simulink model "Test_01"  (R2017b)
settings: Solver=ode45  StartTime=0.0  StopTime=8  RelTol=1e-3  EnableMultiTasking=on
values from neighbouring files (symbols this model uses):
  beta = beta (k)    [Parameter_2M_DFIG_and_BESS.m]
  Cbus = 80e-3    (= 0.08)    [Parameter_2M_DFIG_and_BESS.m]
  cp_opt_abs = abs(max(Cp))    [Parameter_2M_DFIG_and_BESS.m]
  D = 0.1    [Parameter_2M_DFIG_and_BESS.m]
  f = 60    [Parameter_2M_DFIG_and_BESS.m]
  Fs = 1.8    [Parameter_2M_DFIG_and_BESS.m]
  fsw = 4e3    (= 4000)    [Parameter_2M_DFIG_and_BESS.m]
  J = 90    [Parameter_2M_DFIG_and_BESS.m]
  ki_id = (wni^2)*Lr*sigma    (= 491.599501999)    [Parameter_2M_DFIG_and_BESS.m]
  ki_idg = (wnig^2)*Lg    (= 68.6450725305)    [Parameter_2M_DFIG_and_BESS.m]
  ki_iq = ki_id    (= 491.599501999)    [Parameter_2M_DFIG_and_BESS.m]
  ki_iqg = ki_idg    (= 68.6450725305)    [Parameter_2M_DFIG_and_BESS.m]
  ki_v = -300000    [Parameter_2M_DFIG_and_BESS.m]
  kp_id = (2*wni*sigma*Lr)-Rr    (= 0.5771)    [Parameter_2M_DFIG_and_BESS.m]
  kp_idg = (2*wnig*Lg)-Rg    (= 0.364153420404)    [Parameter_2M_DFIG_and_BESS.m]
  kp_iq = kp_id    (= 0.5771)    [Parameter_2M_DFIG_and_BESS.m]
  kp_iqg = kp_idg    (= 0.364153420404)    [Parameter_2M_DFIG_and_BESS.m]
  kp_v = -1000    [Parameter_2M_DFIG_and_BESS.m]
  Kpg = 1/(1.5*Vs*sqrt(2/3))    [Parameter_2M_DFIG_and_BESS.m]
  Kqg = -Kpg    [Parameter_2M_DFIG_and_BESS.m]
  lambda_opt = abs(lambda(posicion))    [Parameter_2M_DFIG_and_BESS.m]
  Lg = 483e-6    (= 0.000483)    [Parameter_2M_DFIG_and_BESS.m]
  Lm = 2.5e-3    (= 0.0025)    [Parameter_2M_DFIG_and_BESS.m]
  Lr = Lm + Lsr    (= 0.002587)    [Parameter_2M_DFIG_and_BESS.m]
  Ls = Lm + Lsi    (= 0.002587)    [Parameter_2M_DFIG_and_BESS.m]
  Lsi = 87e-6    (= 8.7e-05)    [Parameter_2M_DFIG_and_BESS.m]
  N = 100    [Parameter_2M_DFIG_and_BESS.m]
  p = 2    [Parameter_2M_DFIG_and_BESS.m]
  Ps = 2e6    (= 2000000)    [Parameter_2M_DFIG_and_BESS.m]
  Radio = 44    [Parameter_2M_DFIG_and_BESS.m]
  Rg = 20e-6    (= 2e-05)    [Parameter_2M_DFIG_and_BESS.m]
  ro = 1.225    [Parameter_2M_DFIG_and_BESS.m]
  Rr = 2.9e-3    (= 0.0029)    [Parameter_2M_DFIG_and_BESS.m]
  Rs = 2.6e-3    (= 0.0026)    [Parameter_2M_DFIG_and_BESS.m]
  sigma = 1- Lm^2/(Ls*Lr)    (= 0.0661284179513)    [Parameter_2M_DFIG_and_BESS.m]
  Ts = 1/fsw/f    (= 4.16666666667e-06)    [Parameter_2M_DFIG_and_BESS.m]
  Vbus_ref = 1200    [Parameter_2M_DFIG_and_BESS.m]
  Vdc_bat_ref = 1300    [Parameter_2M_DFIG_and_BESS.m]
  Vs = 690    [Parameter_2M_DFIG_and_BESS.m]
undefined symbols (not defined in the file or in its folder): D1, D11, Delta, DiscIntNeverNeededParam, Ion, Lithium
libraries: powerlib x60, powerlib_meascontrol x30, simulink x2, electricdrivelib x1, sps_avr x1
(part 2 of 2)

== system Test_01/BESS 1.0 MW 690 V/Bess Monitor ==
  note: BATTERY STORAGE SYSTEM
  note: Tip Speed Ratio
  note: Charging Power
  note: Discharging Power
  note: Id current control
  Mux{,13..15} (4 alike) : Mux  Inputs=2
  Scope3 : Scope  NumInputPorts=6
  wires:
  [P_bat_ref] -> Mux14/1
  [V_dc_bat] -> Mux/2
  Mux13/1 -> Scope3/2  "Charging Power (W)"
  [P_SOC_ref] -> Mux13/1
  [P_bat] -> Mux14/2, Mux13/2
  [id_bat_ref] -> Mux15/1
  [V_dc_bat_ref] -> Mux/1
  Mux/1 -> Scope3/1  "Vbus* / Vbus (V)"
  [id_bat] -> Mux15/2
  Mux14/1 -> Scope3/3  "Discharging Power (W)"
  [SOC] -> Scope3/5  "SOC (%)"
  [I_dc_bat] -> Scope3/4  "Battery Current (Amp)"
  Mux15/1 -> Scope3/6  "Id*/Id (Amp)"

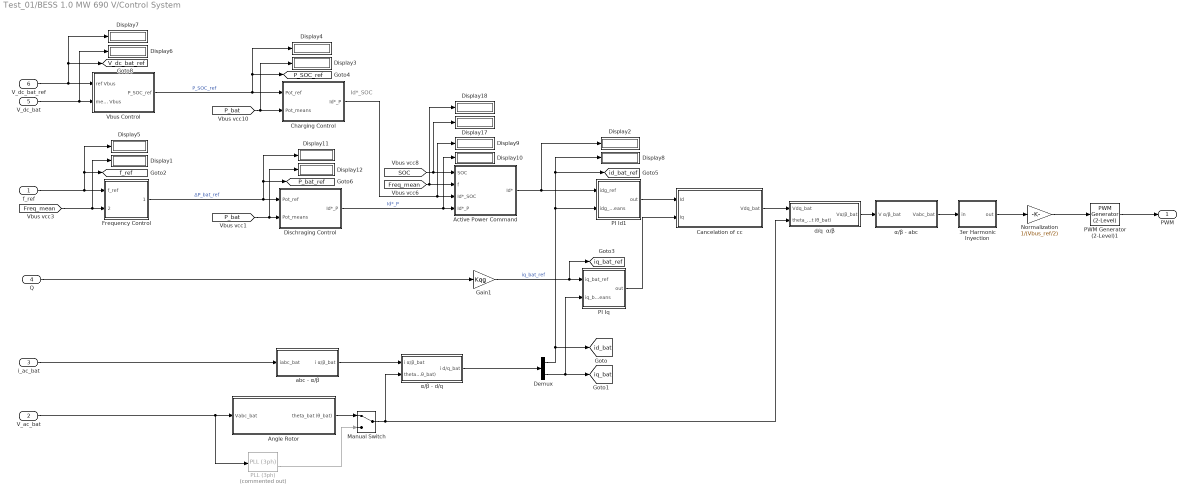
== system Test_01/BESS 1.0 MW 690 V/Control System ==
  note: Id*_SOC
  f_ref : Inport
  "V_ac_bat " : Inport  Port=2
  i_ac_bat : Inport  Port=3
  Q : Inport  Port=4
  V_dc_bat : Inport  Port=5
  V_dc_bat_ref : Inport  Port=6
  " Angle Rotor" : Subsystem
  3er Harmonic Inyection : Subsystem
  Active Power Command : Subsystem
  Cancelation of cc : Subsystem
  Charging Control : Subsystem
  Demux : Demux  Outputs=2
  Dischraging Control : Subsystem
  Display{1..12,17..18} (14 alike) : Display
  Frequency Control : Subsystem
  Gain1 : Gain  Gain=Kqg
  Manual Switch : ManualSwitch
  Normalization : Gain  Gain=1/(Vbus_ref/2)
  PI Id1 : Subsystem
  PI Iq : Subsystem
  PLL (3ph) : powerlib_meascontrol/PLL/PLL (3ph)  Commented=on  Fmin=45  Par_Init=[0, 60]  ParK=[180, 3200, 1]  TcD=1e-4  MaxRateChangeFreq=12  FilterCutOffFreq=25  Ts=0  AGC=on
      link override Model/abc to dq0: Alignment=Aligned with phase A axis
  PWM Generator (2-Level)1 : powerlib_meascontrol/Pulse & Signal Generators/PWM Generator (2-Level)  ModulatorType=Three-phase bridge (6 pulses)  ModulatorMode=Unsynchronized  Fc=fsw  Pc=0  nF=27  MinMax="[ -1  1 ]"  SamplingTechnique=Natural  ModulatingSignals=off  m=0.8  Freq=60  Phase=0  Ts=0  ShowCarrierOutport=off
      settings: SourceProductName=Simscape Power Systems
  Vbus Control : Subsystem
  "abc - α/β  " : Subsystem
  "d/q  α/β " : Subsystem
  α/β - abc : Subsystem
  α/β - d/q : Subsystem
  PWM : Outport
  tag scope: P_SOC_ref=global, P_bat_ref=global, V_dc_bat_ref=global, f_ref=global, id_bat=global, id_bat_ref=global, iq_bat=global, iq_bat_ref=global
  wires:
  PWM Generator (2-Level)1/1 -> PWM/1
  PLL (3ph)/2 -> Manual Switch/2
  α/β - d/q/1(i d/q_bat) -> Demux/1
  Manual Switch/1 -> "d/q  α/β "/2(theta_bat (θ_bat)), α/β - d/q/2(theta_bat (θ_bat))
  " Angle Rotor"/1(theta_bat (θ_bat)) -> Manual Switch/1
  "V_ac_bat "/1 -> PLL (3ph)/1, " Angle Rotor"/1(Vabc_bat)
  α/β - abc/1(Vabc_bat) -> 3er Harmonic Inyection/1(in)
  i_ac_bat/1 -> "abc - α/β  "/1(iabc_bat)
  "d/q  α/β "/1("Vα/β_bat ") -> α/β - abc/1(V α/β_bat)
  "abc - α/β  "/1(i α/β_bat) -> α/β - d/q/1(i α/β_bat)
  3er Harmonic Inyection/1(out) -> Normalization/1
  PI Id1/1(out) -> Cancelation of cc/1(Id)
  PI Iq/1("out ") -> Cancelation of cc/2(Iq)
  Demux/2 -> [iq_bat], PI Iq/2(iq_bat_means)
  Gain1/1 -> [iq_bat_ref], PI Iq/1(iq_bat_ref)  "iq_bat_ref"
  Cancelation of cc/1(" Vdq_bat") -> "d/q  α/β "/1(Vdq_bat)
  Normalization/1 -> PWM Generator (2-Level)1/1
  Frequency Control/1("ΔP_bat_ref ") -> [P_bat_ref], Display11/1, Dischraging Control/1("Pot_ref ")  "ΔP_bat_ref"
  V_dc_bat/1 -> Display6/1, Vbus Control/2("means Vbus ")
  f_ref/1 -> Frequency Control/1(f_ref), [f_ref], Display5/1
  Q/1 -> Gain1/1
  [P_bat] -> Display12/1, Dischraging Control/2("Pot_means ")
  [Freq_mean] -> Display1/1, Frequency Control/2(f_means)
  Demux/1 -> PI Id1/2(idg_means), Display8/1, [id_bat_ref], [id_bat]
  [Freq_mean] -> Active Power Command/2(f), Display18/1
  [SOC] -> Active Power Command/1(SOC), Display17/1
  V_dc_bat_ref/1 -> [V_dc_bat_ref], Display7/1, Vbus Control/1("ref Vbus ")
  Active Power Command/1(Id*) -> Display2/1, PI Id1/1(idg_ref)
  Dischraging Control/1(Id*_P) -> Display10/1, Active Power Command/4(Id*_P)  "Id*_P"
  Charging Control/1(Id*_P) -> Display9/1, Active Power Command/3(Id*_SOC)
  Vbus Control/1(P_SOC_ref) -> [P_SOC_ref], Display4/1, Charging Control/1("Pot_ref ")  "P_SOC_ref"
  [P_bat] -> Charging Control/2("Pot_means "), Display3/1

== system Test_01/BESS 1.0 MW 690 V/Measurement of Power - Frequency ==
  PLL (3ph)1 : powerlib_meascontrol/PLL/PLL (3ph)  Fmin=45  Par_Init=[0, f]  ParK=[180, 3200, 1]  TcD=1e-4  MaxRateChangeFreq=12  FilterCutOffFreq=25  Ts=0  AGC=on
  "Power (3ph, Instantaneous)1" : powerlib_meascontrol/Measurements/Power (3ph, Instantaneous)
      settings: SourceProductName=Simscape Power Systems
  F (Hz) : Outport
  P (W) : Outport  Port=2
  Q (VAR) : Outport  Port=3
  tag scope: Freq_mean=global, P_bat=global, Q_bat=global
  wires:
  [V_ac_bat] -> "Power (3ph, Instantaneous)1"/1, PLL (3ph)1/1
  "Power (3ph, Instantaneous)1"/1 -> P (W)/1, [P_bat]  "Pot"
  PLL (3ph)1/1 -> F (Hz)/1, [Freq_mean]
  [I_ac_bat] -> "Power (3ph, Instantaneous)1"/2
  "Power (3ph, Instantaneous)1"/2 -> Q (VAR)/1, [Q_bat]

== system Test_01/BESS 1.0 MW 690 V/Subsystem1 ==
  In1 : Inport
  Bus Selector : BusSelector  OutputSignals=SOC (%),Current (A),Voltage (V)
  tag scope: I_dc_bat=global, SOC=global, V_dc_bat=global
  wires:
  Bus Selector/3 -> [V_dc_bat]  "<Voltage (V)>"
  Bus Selector/1 -> [SOC]  "<SOC (%)>"
  In1/1 -> Bus Selector/1
  Bus Selector/2 -> [I_dc_bat]  "<Current (A)>"

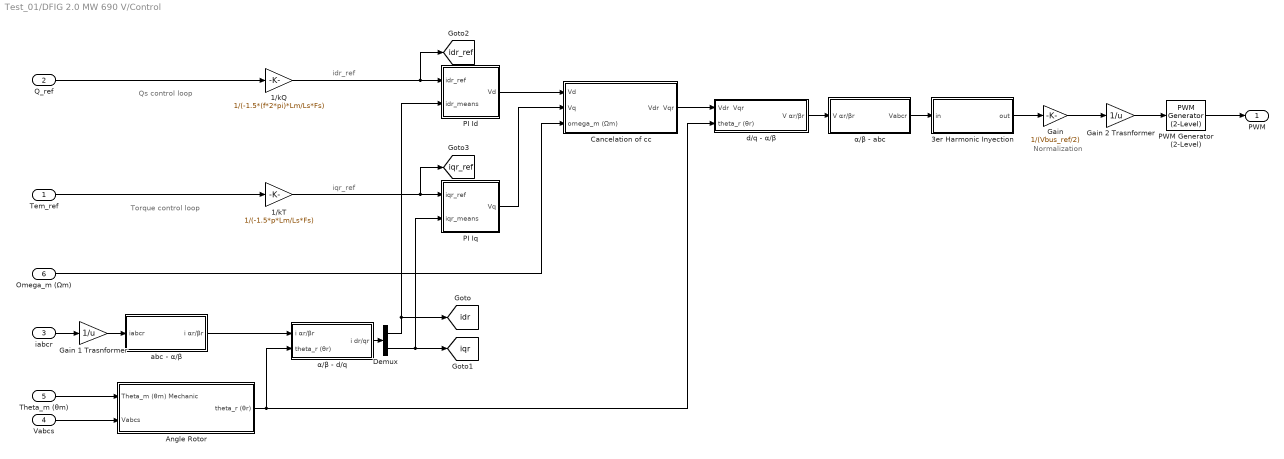
== system Test_01/DFIG 2.0 MW 690 V/Control ==
  note: Normalization
  note: Torque control loop
  note: iqr_ref
  note: idr_ref
  note: Qs control loop
  Tem_ref : Inport
  Q_ref : Inport  Port=2
  iabcr : Inport  Port=3
  Vabcs : Inport  Port=4
  Theta_m (θm) : Inport  Port=5
  "Omega_m (Ωm) " : Inport  Port=6
  " Angle Rotor" : Subsystem
  1/kQ : Gain  Gain=1/(-1.5*(f*2*pi)*Lm/Ls*Fs)
  1/kT : Gain  Gain=1/(-1.5*p*Lm/Ls*Fs)
  3er Harmonic Inyection : Subsystem
  Cancelation of cc : Subsystem
  Demux : Demux  Outputs=2
  Gain : Gain  Gain=1/(Vbus_ref/2)
  Gain 1 Trasnformer : Gain  Gain=1/u
  Gain 2 Trasnformer : Gain  Gain=1/u
  PI Id : Subsystem
  PI Iq : Subsystem
  PWM Generator (2-Level) : powerlib_meascontrol/Pulse & Signal Generators/PWM Generator (2-Level)  ModulatorType=Three-phase bridge (6 pulses)  ModulatorMode=Unsynchronized  Fc=fsw  Pc=0  nF=27  MinMax="[ -1  1 ]"  SamplingTechnique=Natural  ModulatingSignals=off  m=0.8  Freq=60  Phase=0  Ts=0  ShowCarrierOutport=off
      settings: SourceProductName=Simscape Power Systems
  "abc - α/β " : Subsystem
  d/q - α/β : Subsystem
  α/β - abc : Subsystem
  α/β - d/q : Subsystem
  PWM : Outport
  tag scope: idr=global, idr_ref=global, iqr=global, iqr_ref=global
  wires:
  α/β - abc/1(Vabcr) -> 3er Harmonic Inyection/1(in)
  d/q - α/β/1(V αr/βr) -> α/β - abc/1(V αr/βr)
  iabcr/1 -> Gain 1 Trasnformer/1
  "abc - α/β "/1(i αr/βr) -> α/β - d/q/1(i αr/βr)
  3er Harmonic Inyection/1(out) -> Gain/1
  Theta_m (θm)/1 -> " Angle Rotor"/1(Theta_m (θm) Mechanic)
  Vabcs/1 -> " Angle Rotor"/2(Vabcs)
  " Angle Rotor"/1(theta_r (θr)) -> d/q - α/β/2(theta_r (θr)), α/β - d/q/2(theta_r (θr))
  PI Id/1(Vd) -> Cancelation of cc/1(Vd)
  PI Iq/1(Vq) -> Cancelation of cc/2(Vq)
  α/β - d/q/1(i dr/qr) -> Demux/1
  Demux/2 -> PI Iq/2(iqr_means), [iqr]
  Demux/1 -> PI Id/2(idr_means), [idr]
  1/kT/1 -> [iqr_ref], PI Iq/1(iqr_ref)
  Q_ref/1 -> 1/kQ/1
  Cancelation of cc/1(Vdr  Vqr) -> d/q - α/β/1(Vdr  Vqr)
  Gain/1 -> Gain 2 Trasnformer/1
  Gain 1 Trasnformer/1 -> "abc - α/β "/1(iabcr)
  Gain 2 Trasnformer/1 -> PWM Generator (2-Level)/1
  PWM Generator (2-Level)/1 -> PWM/1
  Tem_ref/1 -> 1/kT/1
  "Omega_m (Ωm) "/1 -> Cancelation of cc/3(omega_m (Ωm))
  1/kQ/1 -> [idr_ref], PI Id/1(idr_ref)

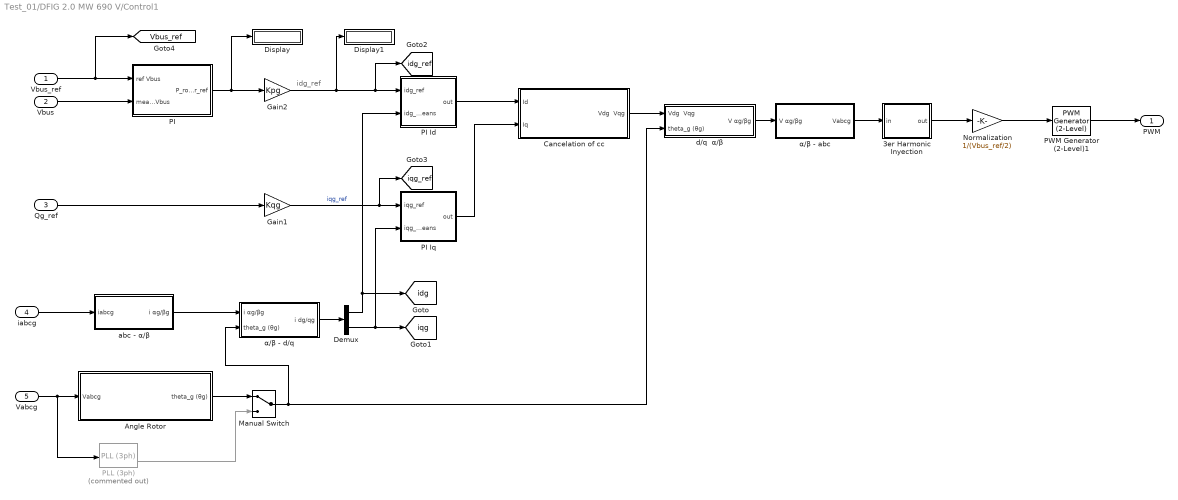
== system Test_01/DFIG 2.0 MW 690 V/Control1 ==
  note: idg_ref
  Vbus_ref : Inport
  Vbus : Inport  Port=2
  Qg_ref : Inport  Port=3
  iabcg : Inport  Port=4
  "Vabcg " : Inport  Port=5
  " Angle Rotor" : Subsystem
  3er Harmonic Inyection : Subsystem
  Cancelation of cc : Subsystem
  Demux : Demux  Outputs=2
  Display : Display
  Display1 : Display
  Gain1 : Gain  Gain=Kqg
  Gain2 : Gain  Gain=Kpg
  Manual Switch : ManualSwitch
  Normalization : Gain  Gain=1/(Vbus_ref/2)
  PI : Subsystem
  PI Id : Subsystem
  PI Iq : Subsystem
  PLL (3ph) : powerlib_meascontrol/PLL/PLL (3ph)  Commented=on  Fmin=45  Par_Init=[0, 60]  ParK=[180, 3200, 1]  TcD=1e-4  MaxRateChangeFreq=12  FilterCutOffFreq=25  Ts=0  AGC=on
      link override Model/abc to dq0: Alignment=Aligned with phase A axis
  PWM Generator (2-Level)1 : powerlib_meascontrol/Pulse & Signal Generators/PWM Generator (2-Level)  ModulatorType=Three-phase bridge (6 pulses)  ModulatorMode=Unsynchronized  Fc=fsw  Pc=0  nF=27  MinMax="[ -1  1 ]"  SamplingTechnique=Natural  ModulatingSignals=off  m=0.8  Freq=60  Phase=0  Ts=0  ShowCarrierOutport=off
      settings: SourceProductName=Simscape Power Systems
  "abc - α/β  " : Subsystem
  "d/q  α/β " : Subsystem
  α/β - abc : Subsystem
  α/β - d/q : Subsystem
  PWM : Outport
  tag scope: Vbus_ref=global, idg=global, idg_ref=global, iqg=global, iqg_ref=global
  wires:
  Normalization/1 -> PWM Generator (2-Level)1/1
  Cancelation of cc/1(Vdg  Vqg) -> "d/q  α/β "/1(Vdg  Vqg)
  Gain1/1 -> PI Iq/1(iqg_ref), [iqg_ref]  "iqg_ref"
  Demux/1 -> PI Id/2(idg_means), [idg]
  Demux/2 -> PI Iq/2(iqg_means), [iqg]
  PI Iq/1(out) -> Cancelation of cc/2(Iq)
  PI Id/1(out) -> Cancelation of cc/1(Id)
  3er Harmonic Inyection/1(out) -> Normalization/1
  "abc - α/β  "/1(i αg/βg) -> α/β - d/q/1(i αg/βg)
  "d/q  α/β "/1(V αg/βg) -> α/β - abc/1(V αg/βg)
  iabcg/1 -> "abc - α/β  "/1(iabcg)
  Vbus_ref/1 -> [Vbus_ref], PI/1("ref Vbus ")
  Gain2/1 -> Display1/1, [idg_ref], PI Id/1(idg_ref)
  Vbus/1 -> PI/2("means Vbus ")
  Qg_ref/1 -> Gain1/1
  α/β - abc/1(Vabcg) -> 3er Harmonic Inyection/1(in)
  "Vabcg "/1 -> " Angle Rotor"/1("Vabcg "), PLL (3ph)/1
  PI/1(P_rotor_ref) -> Display/1, Gain2/1
  " Angle Rotor"/1(theta_g (θg)) -> Manual Switch/1
  Manual Switch/1 -> "d/q  α/β "/2(theta_g (θg)), α/β - d/q/2(theta_g (θg))
  α/β - d/q/1(i dg/qg) -> Demux/1
  PLL (3ph)/2 -> Manual Switch/2
  PWM Generator (2-Level)1/1 -> PWM/1

== system Test_01/DFIG 2.0 MW 690 V/MPPT ==
  note: Zone 2: MPPT with Vw 5 - 11
  Omega_m : Inport
  Display1 : Display
  Display2 : Display
  Gearbox Ratio Generator Torque (-)1 : Gain  Gain=-1/N
  Gearbox Ratio1 : Gain  Gain=1/N
  Kopt : Gain  Gain=0.5*ro*pi*(Radio)^5/(lambda_opt)^3*cp_opt_abs
  Product2 : Product  Inputs=**  SaturateOnIntegerOverflow=on  InputSameDT=on  OutDataTypeStr=Inherit: Same as first input
  omega^2 : Fcn  Expr=(u[1])^2
  Tem_ref : Outport
  "Pot_ref " : Outport  Port=2
  wires:
  Gearbox Ratio1/1 -> Product2/2, omega^2/1
  omega^2/1 -> Kopt/1
  Kopt/1 -> Product2/1, Gearbox Ratio Generator Torque (-)1/1
  Product2/1 -> "Pot_ref "/1, Display1/1  "Pt"
  Gearbox Ratio Generator Torque (-)1/1 -> Display2/1, Tem_ref/1
  Omega_m/1 -> Gearbox Ratio1/1

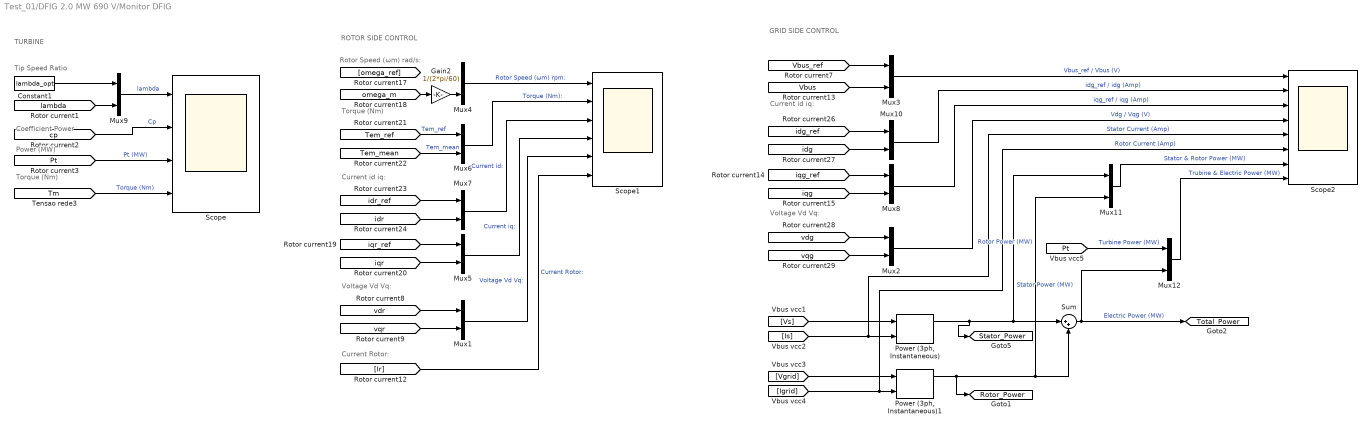
== system Test_01/DFIG 2.0 MW 690 V/Monitor DFIG ==
  note: ROTOR SIDE CONTROL
  note: Torque (Nm)
  note: Current id iq:
  note: Rotor Speed (ωm) rad/s:
  note: Voltage Vd Vq:
  note: TURBINE
  note: Torque (Nm)
  note: Power (MW)
  note: Coefficient Power
  note: Tip Speed Ratio
  note: GRID SIDE CONTROL
  note: Current id iq:
  note: Voltage Vd Vq:
  note: Current Rotor:
  Constant1 : Constant  Value=lambda_opt
  Gain2 : Gain  Gain=1/(2*pi/60)
  Mux{1..12} (12 alike) : Mux  Inputs=2
  "Power (3ph, Instantaneous)" : powerlib_meascontrol/Measurements/Power (3ph, Instantaneous)
      settings: SourceProductName=Simscape Power Systems
  "Power (3ph, Instantaneous)1" : powerlib_meascontrol/Measurements/Power (3ph, Instantaneous)
      settings: SourceProductName=Simscape Power Systems
  Scope : Scope  NumInputPorts=4
  Scope1 : Scope  NumInputPorts=6
  Scope2 : Scope  NumInputPorts=8
  Sum : Sum  Inputs=|++
  tag scope: Rotor_Power=global, Stator_Power=global, Total_Power=global
  wires:
  [iqr_ref] -> Mux5/1
  [iqr] -> Mux5/2
  [idr] -> Mux7/2
  [idr_ref] -> Mux7/1
  [vdr] -> Mux1/1
  [vqr] -> Mux1/2
  [vqg] -> Mux2/2
  [vdg] -> Mux2/1
  [idg_ref] -> Mux10/1
  [idg] -> Mux10/2
  [iqg] -> Mux8/2
  [iqg_ref] -> Mux8/1
  [Tem_ref] -> Mux6/1  "Tem_ref"
  [Vbus] -> Mux3/2
  [Vbus_ref] -> Mux3/1
  [cp] -> Scope/2  "Cp"
  [Pt] -> Scope/3  "Pt (MW)"
  [Tm] -> Scope/4  "Torque (Nm)"
  Mux4/1 -> Scope1/1  "Rotor Speed (ωm) rpm:"
  Mux6/1 -> Scope1/2  "Torque (Nm):"
  Mux7/1 -> Scope1/3  "Current id:"
  Mux5/1 -> Scope1/4  "Current iq:"
  Mux1/1 -> Scope1/5  "Voltage Vd Vq:"
  [Ir] -> Scope1/6  "Current Rotor:"
  [omega_m] -> Gain2/1
  Gain2/1 -> Mux4/2
  Mux3/1 -> Scope2/1  "Vbus_ref / Vbus (V)"
  Mux10/1 -> Scope2/2  "idg_ref / idg (Amp)"
  Mux8/1 -> Scope2/3  "iqg_ref / iqg (Amp)"
  Mux2/1 -> Scope2/4  "Vdg / Vqg (V)"
  [lambda] -> Mux9/2
  Constant1/1 -> Mux9/1
  Mux9/1 -> Scope/1  "lambda"
  [Tem_mean] -> Mux6/2  "Tem_mean"
  [Vs] -> "Power (3ph, Instantaneous)"/1
  [Vgrid] -> "Power (3ph, Instantaneous)1"/1
  [Igrid] -> "Power (3ph, Instantaneous)1"/2, Scope2/6  "Rotor Current (Amp)"
  [Is] -> "Power (3ph, Instantaneous)"/2, Scope2/5  "Stator Current (Amp)"
  "Power (3ph, Instantaneous)"/1 -> [Stator_Power], Mux11/1, Sum/1  "Stator Power (MW)"
  "Power (3ph, Instantaneous)1"/1 -> [Rotor_Power], Sum/2, Mux11/2  "Rotor Power (MW)"
  Sum/1 -> [Total_Power], Mux12/2  "Electric Power (MW)"
  Mux11/1 -> Scope2/7  "Stator & Rotor Power (MW)"
  [Pt] -> Mux12/1  "Turbine Power (MW)"
  Mux12/1 -> Scope2/8  "Trubine & Electric Power (MW)"

== system Test_01/DFIG 2.0 MW 690 V/Subsystem ==
  In1 : Inport
  Bus Selector : BusSelector  OutputSignals=Mechanical.Rotor angle thetam (rad),Mechanical.Rotor speed (wm),Mechanical.Electromagnetic torque Te (N*m)
  tag scope: Tem_mean=global, omega_m=global, tita_m=global
  wires:
  Bus Selector/2 -> [omega_m]  "<Rotor speed (wm)>"
  In1/1 -> Bus Selector/1
  Bus Selector/1 -> [tita_m]  "<Rotor angle thetam (rad)>"
  Bus Selector/3 -> [Tem_mean]  "<Electromagnetic torque Te (N*m)>"

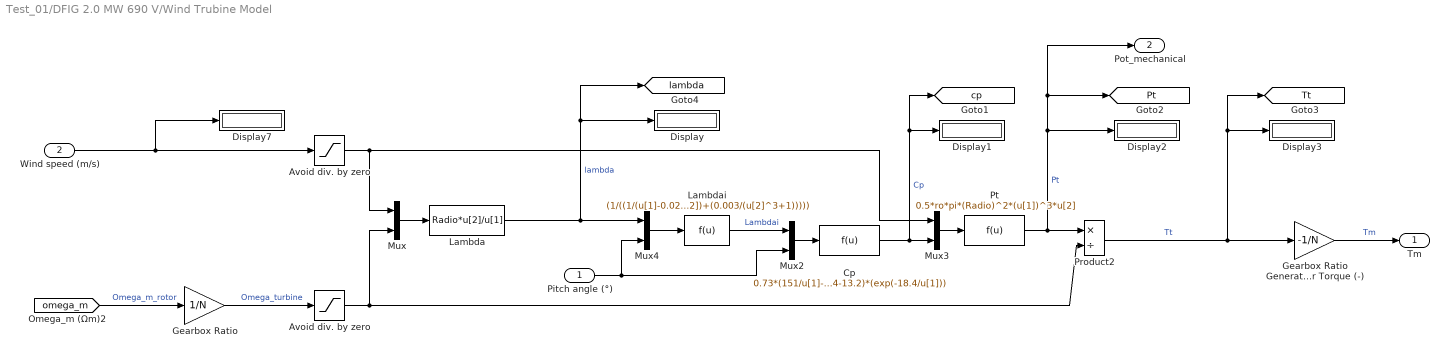
== system Test_01/DFIG 2.0 MW 690 V/Wind Trubine Model ==
  Pitch angle (°) : Inport
  Wind speed (m/s) : Inport  Port=2
  Avoid div. by zero : Saturate  UpperLimit=inf  LowerLimit=eps
  "Avoid div. by zero " : Saturate  UpperLimit=inf  LowerLimit=eps
  Cp : Fcn  Expr=0.73*(151/u[1]-0.58*u[2]-0.002*u[2]^2.14-13.2)*(exp(-18.4/u[1]))
  Display{,1..3,7} (5 alike) : Display
  Gearbox Ratio : Gain  Gain=1/N
  Gearbox Ratio Generator Torque (-) : Gain  Gain=-1/N
  Lambda : Fcn  Expr=Radio*u[2]/u[1]
  Lambdai : Fcn  Expr=(1/((1/(u[1]-0.02*u[2])+(0.003/(u[2]^3+1)))))
  Mux{,2..4} (4 alike) : Mux  Inputs=2
  Product2 : Product  Inputs=*/  SaturateOnIntegerOverflow=on  InputSameDT=on  OutDataTypeStr=Inherit: Same as first input
  Pt : Fcn  Expr=0.5*ro*pi*(Radio)^2*(u[1])^3*u[2]
  Tm : Outport
  Pot_mechanical : Outport  Port=2
  tag scope: Pt=global, Tt=global, cp=global, lambda=global
  wires:
  "Avoid div. by zero "/1 -> Product2/2, Mux/2
  Avoid div. by zero/1 -> Mux/1, Mux3/1
  [omega_m] -> Gearbox Ratio/1  "Omega_m_rotor"
  Mux3/1 -> Pt/1
  Cp/1 -> Display1/1, [cp], Mux3/2  "Cp"
  Mux/1 -> Lambda/1
  Mux2/1 -> Cp/1
  Product2/1 -> Display3/1, [Tt], Gearbox Ratio Generator Torque (-)/1  "Tt"
  Pt/1 -> Display2/1, Pot_mechanical/1, [Pt], Product2/1  "Pt"
  Gearbox Ratio/1 -> "Avoid div. by zero "/1  "Omega_turbine"
  Wind speed (m/s)/1 -> Display7/1, Avoid div. by zero/1
  Lambdai/1 -> Mux2/1  "Lambdai"
  Mux4/1 -> Lambdai/1
  Gearbox Ratio Generator Torque (-)/1 -> Tm/1  "Tm"
  Pitch angle (°)/1 -> Mux2/2, Mux4/2
  Lambda/1 -> Display/1, [lambda], Mux4/1  "lambda"

== system Test_01/Subsystem/Measurement of Power - Frequency1 ==
  PLL (3ph)1 : powerlib_meascontrol/PLL/PLL (3ph)  Fmin=45  Par_Init=[0, f]  ParK=[180, 3200, 1]  TcD=1e-4  MaxRateChangeFreq=12  FilterCutOffFreq=25  Ts=0  AGC=on
  "Power (3ph, Instantaneous)1" : powerlib_meascontrol/Measurements/Power (3ph, Instantaneous)
      settings: SourceProductName=Simscape Power Systems
  F (Hz) : Outport
  P (W) : Outport  Port=2
  wires:
  [I_ac_syn_low1] -> "Power (3ph, Instantaneous)1"/2
  PLL (3ph)1/1 -> F (Hz)/1
  "Power (3ph, Instantaneous)1"/1 -> P (W)/1  "Pot"
  [V_ac_syn_low1] -> PLL (3ph)1/1, "Power (3ph, Instantaneous)1"/1

== system Test_01/Subsystem/Measurement of Power - Frequency2 ==
  PLL (3ph)1 : powerlib_meascontrol/PLL/PLL (3ph)  Fmin=45  Par_Init=[0, f]  ParK=[180, 3200, 1]  TcD=1e-4  MaxRateChangeFreq=12  FilterCutOffFreq=25  Ts=0  AGC=on
  "Power (3ph, Instantaneous)1" : powerlib_meascontrol/Measurements/Power (3ph, Instantaneous)
      settings: SourceProductName=Simscape Power Systems
  F (Hz) : Outport
  P (W) : Outport  Port=2
  wires:
  [I_ac_syn_low2] -> "Power (3ph, Instantaneous)1"/2
  PLL (3ph)1/1 -> F (Hz)/1
  "Power (3ph, Instantaneous)1"/1 -> P (W)/1  "Pot"
  [V_ac_syn_low2] -> PLL (3ph)1/1, "Power (3ph, Instantaneous)1"/1

== system Test_01/BESS 1.0 MW 690 V/Control System/ Angle Rotor ==
  note: V α/β_bat
  Vabc_bat : Inport
  " abc - αβ " : Subsystem
  Demux : Demux  Outputs=2
  θv=tan^(-1) (Vβ/Vα) : Trigonometry  Operator=atan2
  theta_bat (θ_bat) : Outport
  wires:
  θv=tan^(-1) (Vβ/Vα)/1 -> theta_bat (θ_bat)/1
  Vabc_bat/1 -> " abc - αβ "/1(Vabc_bat)
  Demux/2 -> θv=tan^(-1) (Vβ/Vα)/1
  Demux/1 -> θv=tan^(-1) (Vβ/Vα)/2
  " abc - αβ "/1("V α/β_bat ") -> Demux/1

== system Test_01/BESS 1.0 MW 690 V/Control System/3er Harmonic Inyection ==
  in : Inport
  Gain : Gain  Gain=-0.5
  MinMax : MinMax
  MinMax1 : MinMax  Function=max
  Scope : Scope
  Sum : Sum  Inputs=|++
  Sum1 : Sum  Inputs=|++
  out : Outport
  wires:
  in/1 -> Sum1/1, MinMax1/1, MinMax/1
  MinMax/1 -> Sum/1
  MinMax1/1 -> Sum/2
  Sum1/1 -> out/1
  Sum/1 -> Gain/1
  Gain/1 -> Scope/1, Sum1/2

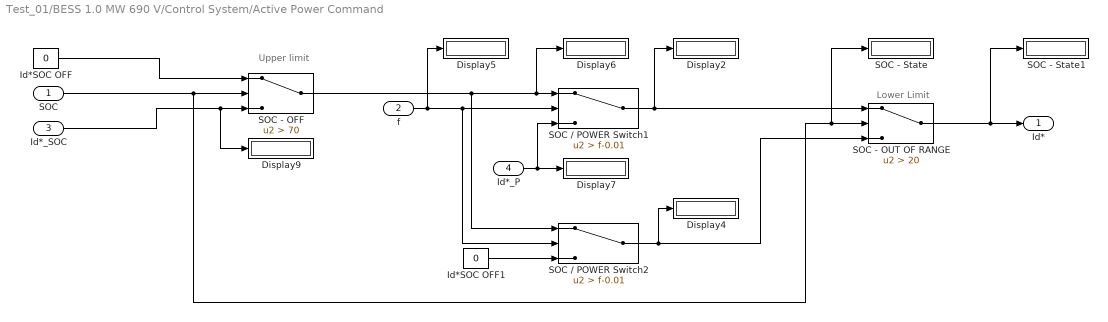
== system Test_01/BESS 1.0 MW 690 V/Control System/Active Power Command ==
  note: Lower Limit
  note: Upper limit
  SOC : Inport
  f : Inport  Port=2
  Id*_SOC : Inport  Port=3
  Id*_P : Inport  Port=4
  Display{2,4..7,9} (6 alike) : Display
  Id*SOC OFF : Constant  Value=0
  Id*SOC OFF1 : Constant  Value=0
  SOC - OFF : Switch  Criteria=u2 > Threshold  Threshold=70
  SOC - OUT OF RANGE : Switch  Criteria=u2 > Threshold  Threshold=20
  SOC - State : Display
  SOC - State1 : Display
  SOC / POWER Switch1 : Switch  Criteria=u2 > Threshold  Threshold=f-0.01
  SOC / POWER Switch2 : Switch  Criteria=u2 > Threshold  Threshold=f-0.01
  Id* : Outport
  wires:
  SOC / POWER Switch1/1 -> SOC - OUT OF RANGE/1, Display2/1
  f/1 -> Display5/1, SOC / POWER Switch2/2, SOC / POWER Switch1/2
  Id*_P/1 -> SOC / POWER Switch1/3, Display7/1
  SOC - OFF/1 -> SOC / POWER Switch2/1, SOC / POWER Switch1/1, Display6/1
  Id*SOC OFF/1 -> SOC - OFF/1
  Id*_SOC/1 -> Display9/1, SOC - OFF/3
  SOC / POWER Switch2/1 -> Display4/1, SOC - OUT OF RANGE/3
  SOC - OUT OF RANGE/1 -> SOC - State1/1, Id*/1
  Id*SOC OFF1/1 -> SOC / POWER Switch2/3
  SOC/1 -> SOC - State/1, SOC - OUT OF RANGE/2, SOC - OFF/2

== system Test_01/BESS 1.0 MW 690 V/Control System/Cancelation of cc ==
  Id : Inport
  Iq : Inport  Port=2
  Display : Display
  Fcn : Fcn  Expr=u[1]-u[4]*Lg*(2*pi*f)
  Fcn1 : Fcn  Expr=u[2]+u[3]*Lg*(2*pi*f)
  Mux : Mux  Inputs=2
  Mux1 : Mux
  " Vdq_bat" : Outport
  tag scope: vd_bat=global, vq_bat=global
  wires:
  Mux/1 -> " Vdq_bat"/1
  Fcn/1 -> [vd_bat], Display/1, Mux/1
  Fcn1/1 -> [vq_bat], Mux/2
  Id/1 -> Mux1/1
  Iq/1 -> Mux1/2
  Mux1/1 -> Fcn1/1, Fcn/1
  [id_bat] -> Mux1/3
  [iq_bat] -> Mux1/4

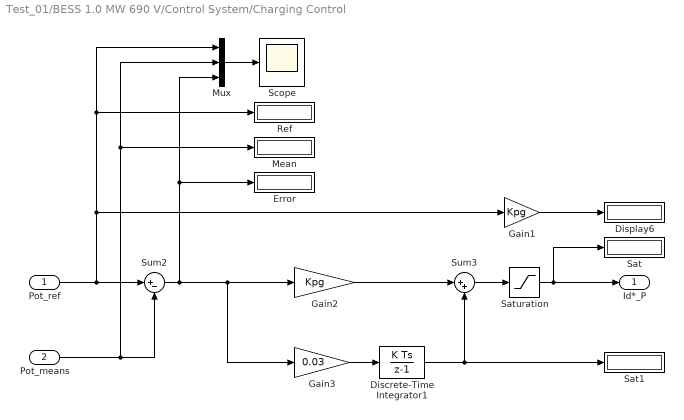
== system Test_01/BESS 1.0 MW 690 V/Control System/Charging Control ==
  "Pot_ref " : Inport
  "Pot_means " : Inport  Port=2
  Discrete-Time Integrator1 : DiscreteIntegrator  gainval=1  SampleTime=1/fsw  LimitOutput=on  UpperSaturationLimit=1200  LowerSaturationLimit=-1200  ICPrevOutput=DiscIntNeverNeededParam  ICPrevScaledInput=DiscIntNeverNeededParam
  Display6 : Display
  Error : Display
  Gain1 : Gain  Gain=Kpg
  Gain2 : Gain  Gain=Kpg
  Gain3 : Gain  Gain=0.03
  Mean : Display
  Mux : Mux  Inputs=3
  Ref : Display
  Sat : Display
  Sat1 : Display
  Saturation : Saturate  UpperLimit=1200  LowerLimit=-1200
  Scope : Scope
  Sum2 : Sum  Inputs=|+-
  Sum3 : Sum  Inputs=|++
  Id*_P : Outport
  wires:
  Sum2/1 -> Error/1, Mux/3, Gain2/1, Gain3/1
  Gain1/1 -> Display6/1
  Gain2/1 -> Sum3/1
  Sum3/1 -> Saturation/1
  Gain3/1 -> Discrete-Time Integrator1/1
  Discrete-Time Integrator1/1 -> Sat1/1, Sum3/2
  Mux/1 -> Scope/1
  "Pot_ref "/1 -> Mux/1, Ref/1, Gain1/1, Sum2/1
  "Pot_means "/1 -> Mux/2, Mean/1, Sum2/2
  Saturation/1 -> Sat/1, Id*_P/1

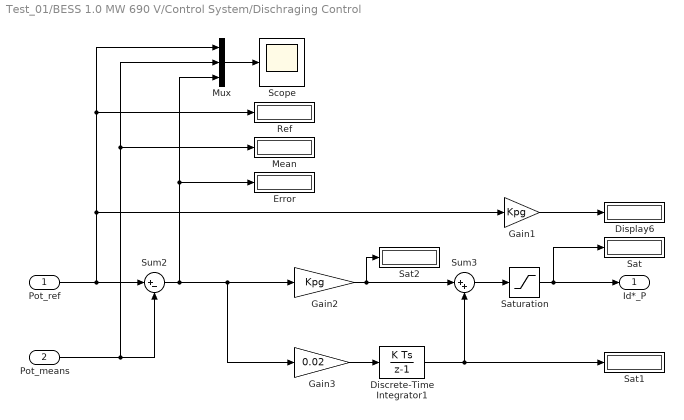
== system Test_01/BESS 1.0 MW 690 V/Control System/Dischraging Control ==
  "Pot_ref " : Inport
  "Pot_means " : Inport  Port=2
  Discrete-Time Integrator1 : DiscreteIntegrator  gainval=1  SampleTime=1/fsw  LimitOutput=on  UpperSaturationLimit=1850  LowerSaturationLimit=-1850  ICPrevOutput=DiscIntNeverNeededParam  ICPrevScaledInput=DiscIntNeverNeededParam
  Display6 : Display
  Error : Display
  Gain1 : Gain  Gain=Kpg
  Gain2 : Gain  Gain=Kpg
  Gain3 : Gain  Gain=0.02
  Mean : Display
  Mux : Mux  Inputs=3
  Ref : Display
  Sat : Display
  Sat1 : Display
  Sat2 : Display
  Saturation : Saturate  UpperLimit=1850  LowerLimit=-1850
  Scope : Scope
  Sum2 : Sum  Inputs=|+-
  Sum3 : Sum  Inputs=|++
  Id*_P : Outport
  wires:
  Saturation/1 -> Id*_P/1, Sat/1
  "Pot_means "/1 -> Sum2/2, Mean/1, Mux/2
  "Pot_ref "/1 -> Sum2/1, Gain1/1, Ref/1, Mux/1
  Mux/1 -> Scope/1
  Discrete-Time Integrator1/1 -> Sum3/2, Sat1/1
  Gain3/1 -> Discrete-Time Integrator1/1
  Sum3/1 -> Saturation/1
  Gain2/1 -> Sat2/1, Sum3/1
  Gain1/1 -> Display6/1
  Sum2/1 -> Gain3/1, Gain2/1, Mux/3, Error/1

== system Test_01/BESS 1.0 MW 690 V/Control System/Frequency Control ==
  note: Δf = f_ref - f_means
  note: R = (Δf/fo)/(ΔP/Po)*100
  note: ΔP = 1/fo* Δf * 1/R * 100 * Po
  f_ref : Inport
  f_means : Inport  Port=2
  Dead Zone : DeadZone  LowerValue=-0.12*1/f  UpperValue=0.02*1/f  SaturateOnIntegerOverflow=on
  Droop : Gain  Gain=1/(2.5)*100
  Error : Display
  Mean : Display
  Mux : Mux  Inputs=3
  Ref : Display
  Saturation : Saturate  UpperLimit=1  LowerLimit=0
  Scope : Scope
  Sum : Sum  Inputs=|+-
  "pu_Pot " : Gain  Gain=2.6e6
  pu_f : Gain  Gain=1/f
  pu_f2 : Gain  Gain=1/f
  ΔP_bat_ref : Display
  ΔP_bat_ref1 : Display
  "ΔP_bat_ref " : Outport
  wires:
  Mux/1 -> Scope/1
  Sum/1 -> Mux/3, Error/1, Dead Zone/1
  f_ref/1 -> pu_f/1
  f_means/1 -> pu_f2/1
  Droop/1 -> Saturation/1
  Dead Zone/1 -> Droop/1
  Saturation/1 -> ΔP_bat_ref1/1, "pu_Pot "/1
  pu_f/1 -> Sum/1, Mux/1, Ref/1
  pu_f2/1 -> Sum/2, Mux/2, Mean/1
  "pu_Pot "/1 -> ΔP_bat_ref/1, "ΔP_bat_ref "/1

== system Test_01/BESS 1.0 MW 690 V/Control System/PI Id1 ==
  idg_ref : Inport
  idg_means : Inport  Port=2
  Discrete-Time Integrator : DiscreteIntegrator  SampleTime=1/fsw  LimitOutput=on  UpperSaturationLimit=Vbus_ref/sqrt(3)*5  LowerSaturationLimit=-Vbus_ref/sqrt(3)*5  ICPrevOutput=DiscIntNeverNeededParam  ICPrevScaledInput=DiscIntNeverNeededParam
  Error : Display
  Gain : Gain  Gain=kp_idg
  Gain1 : Gain  Gain=ki_idg*0.35
  Mean : Display
  Mux : Mux  Inputs=3
  Ref : Display
  Sat : Display
  Sat 1 : Display
  Saturation : Saturate  UpperLimit=Vbus_ref/sqrt(3)*6  LowerLimit=-Vbus_ref/sqrt(3)*6
  Scope : Scope
  Sum : Sum  Inputs=|+-
  Sum1 : Sum  Inputs=|++
  out : Outport
  wires:
  Saturation/1 -> Sat/1, out/1
  Sum1/1 -> Saturation/1
  Discrete-Time Integrator/1 -> Sat 1/1, Sum1/2
  Gain1/1 -> Discrete-Time Integrator/1
  Gain/1 -> Sum1/1
  idg_means/1 -> Mean/1, Mux/2, Sum/2
  idg_ref/1 -> Ref/1, Mux/1, Sum/1
  Sum/1 -> Gain/1, Gain1/1, Mux/3, Error/1
  Mux/1 -> Scope/1

== system Test_01/BESS 1.0 MW 690 V/Control System/PI Iq ==
  iq_bat_ref : Inport
  iq_bat_means : Inport  Port=2
  Discrete-Time Integrator : DiscreteIntegrator  SampleTime=1/fsw  LimitOutput=on  UpperSaturationLimit=Vbus_ref/sqrt(3)  LowerSaturationLimit=-Vbus_ref/sqrt(3)  ICPrevOutput=DiscIntNeverNeededParam  ICPrevScaledInput=DiscIntNeverNeededParam
  Error : Display
  Gain : Gain  Gain=kp_iqg
  Gain1 : Gain  Gain=ki_iqg
  Mean : Display
  Mux : Mux  Inputs=3
  Ref : Display
  Sat : Display
  Sat 1 : Display
  Saturation : Saturate  UpperLimit=Vbus_ref/sqrt(3)  LowerLimit=-Vbus_ref/sqrt(3)
  Scope : Scope
  Sum : Sum  Inputs=|+-
  Sum1 : Sum  Inputs=|++
  "out " : Outport
  wires:
  Mux/1 -> Scope/1
  Sum/1 -> Gain1/1, Gain/1, Error/1, Mux/3
  iq_bat_ref/1 -> Mux/1, Ref/1, Sum/1
  iq_bat_means/1 -> Mux/2, Mean/1, Sum/2
  Saturation/1 -> "out "/1, Sat/1
  Gain/1 -> Sum1/1
  Gain1/1 -> Discrete-Time Integrator/1
  Discrete-Time Integrator/1 -> Sum1/2, Sat 1/1
  Sum1/1 -> Saturation/1

== system Test_01/BESS 1.0 MW 690 V/Control System/Vbus Control ==
  note: signal
  note: reference
  "ref Vbus " : Inport
  "means Vbus " : Inport  Port=2
  Discrete-Time Integrator1 : DiscreteIntegrator  SampleTime=1/fsw  LimitOutput=on  UpperSaturationLimit=0.5e6  LowerSaturationLimit=-0.5e6  ICPrevOutput=DiscIntNeverNeededParam  ICPrevScaledInput=DiscIntNeverNeededParam
  Error : Display
  Gain2 : Gain  Gain=-1000
  Gain3 : Gain  Gain=-300000
  Mean : Display
  Mux : Mux  Inputs=3
  Ref : Display
  Sat : Display
  Sat 1 : Display
  Saturation1 : Saturate  UpperLimit=0.5e6  LowerLimit=-0.5e6
  Scope : Scope
  Sum2 : Sum  Inputs=|+-
  Sum3 : Sum  Inputs=|++
  P_SOC_ref : Outport
  wires:
  Discrete-Time Integrator1/1 -> Sat 1/1, Sum3/2
  Gain3/1 -> Discrete-Time Integrator1/1
  Sum3/1 -> Saturation1/1
  Gain2/1 -> Sum3/1
  Saturation1/1 -> Sat/1, P_SOC_ref/1
  "means Vbus "/1 -> Sum2/2, Mean/1, Mux/2
  "ref Vbus "/1 -> Sum2/1, Ref/1, Mux/1
  Sum2/1 -> Gain2/1, Gain3/1, Mux/3, Error/1
  Mux/1 -> Scope/1

== system Test_01/BESS 1.0 MW 690 V/Control System/abc - α//β   ==
  note: iβ_bat
  note: iα_bat
  iabc_bat : Inport
  Fcn : Fcn  Expr=2/3*(u[1]-u[2]/2-u[3]/2)
  Fcn1 : Fcn  Expr=2/3*(u[2]*(sqrt(3)/2)-u[3]*(sqrt(3)/2))
  Mux : Mux  Inputs=2
  i α/β_bat : Outport
  wires:
  Mux/1 -> i α/β_bat/1
  iabc_bat/1 -> Fcn1/1, Fcn/1
  Fcn/1 -> Mux/1
  Fcn1/1 -> Mux/2

== system Test_01/BESS 1.0 MW 690 V/Control System/d//q  α//β  ==
  Vdq_bat : Inport
  theta_bat (θ_bat) : Inport  Port=2
  Fcn : Fcn  Expr=u(1)*cos(u[3])-u[2]*sin(u[3])
  Fcn1 : Fcn  Expr=u(1)*sin(u[3])+u[2]*cos(u[3])
  Mux : Mux  Inputs=2
  Mux1 : Mux  Inputs=2
  "Vα/β_bat " : Outport
  wires:
  Mux/1 -> "Vα/β_bat "/1
  Fcn/1 -> Mux/1
  Fcn1/1 -> Mux/2
  Vdq_bat/1 -> Mux1/1
  theta_bat (θ_bat)/1 -> Mux1/2
  Mux1/1 -> Fcn/1, Fcn1/1

== system Test_01/BESS 1.0 MW 690 V/Control System/α//β - abc ==
  V α/β_bat : Inport
  Fcn : Fcn  Expr=u(1)
  Fcn1 : Fcn  Expr=-(u[1]/2)+u[2]*(sqrt(3)/2)
  Fcn2 : Fcn  Expr=-(u[1]/2)-u[2]*(sqrt(3)/2)
  Mux : Mux  Inputs=3
  Vabc_bat : Outport
  wires:
  Mux/1 -> Vabc_bat/1
  V α/β_bat/1 -> Fcn2/1, Fcn1/1, Fcn/1
  Fcn/1 -> Mux/1
  Fcn1/1 -> Mux/2
  Fcn2/1 -> Mux/3

== system Test_01/BESS 1.0 MW 690 V/Control System/α//β - d//q ==
  i α/β_bat : Inport
  theta_bat (θ_bat) : Inport  Port=2
  Fcn : Fcn  Expr=u(1)*cos(u[3])+u[2]*sin(u[3])
  Fcn1 : Fcn  Expr=-u(1)*sin(u[3])+u[2]*cos(u[3])
  Mux : Mux  Inputs=2
  Mux1 : Mux  Inputs=2
  i d/q_bat : Outport
  wires:
  Mux/1 -> i d/q_bat/1
  Fcn/1 -> Mux/1
  Fcn1/1 -> Mux/2
  i α/β_bat/1 -> Mux1/1
  theta_bat (θ_bat)/1 -> Mux1/2
  Mux1/1 -> Fcn1/1, Fcn/1

== system Test_01/DFIG 2.0 MW 690 V/Control/ Angle Rotor ==
  note: Theta_m (θm)
      | Electric
  note: theta_V θv
  note: The stator reference frame (α - β) is a stationary
      | reference frame.
  note: The relation between the mechanical angle of the shaft and the
      | electrical angle depends on the pole pairs of the machine:
      |
      | θm (electrical) = Pole * θm (mechanical)
  note: theta_s (θs)
  note: Vαs/βs
  note: θs=θv-90°
  note: θs=θr+θm
      | θr=θs-θm
  note: Vector control of the DFIM is performed in a synchronously rotating dq frame, in which the d-axis is aligned, in this case, with the stator flux space vector
  Theta_m (θm) Mechanic : Inport
  Vabcs : Inport  Port=2
  "Clarke: abc - αβ " : Subsystem
  Constant : Constant  Value=pi/2
  Demux : Demux  Outputs=2
  Manual Switch1 : ManualSwitch  CurrentSetting=0
  PLL (3ph)1 : powerlib_meascontrol/PLL/PLL (3ph)  Commented=on  Fmin=45  Par_Init=[0, 60]  ParK=[180, 3200, 1]  TcD=1e-4  MaxRateChangeFreq=12  FilterCutOffFreq=25  Ts=0  AGC=on
      link override Model/abc to dq0: Alignment=Aligned with phase A axis
  Pole Pairs : Gain  Gain=p
  Sum : Sum  Inputs=|+-
  Sum1 : Sum  Inputs=|+-
  θv=tan^(-1) (Vβ/Vα) : Trigonometry  Operator=atan2
  theta_r (θr) : Outport
  wires:
  Vabcs/1 -> PLL (3ph)1/1, "Clarke: abc - αβ "/1(Vabc)
  Demux/2 -> θv=tan^(-1) (Vβ/Vα)/1
  Demux/1 -> θv=tan^(-1) (Vβ/Vα)/2
  "Clarke: abc - αβ "/1("Vαs/βs ") -> Demux/1
  Constant/1 -> Sum/2
  Theta_m (θm) Mechanic/1 -> Pole Pairs/1
  Sum/1 -> Sum1/1
  Sum1/1 -> theta_r (θr)/1
  Pole Pairs/1 -> Sum1/2
  Manual Switch1/1 -> Sum/1
  θv=tan^(-1) (Vβ/Vα)/1 -> Manual Switch1/2
  PLL (3ph)1/2 -> Manual Switch1/1

== system Test_01/DFIG 2.0 MW 690 V/Control/3er Harmonic Inyection ==
  in : Inport
  Gain : Gain  Gain=-0.5
  MinMax : MinMax
  MinMax1 : MinMax  Function=max
  Scope : Scope
  Sum : Sum  Inputs=|++
  Sum1 : Sum  Inputs=|++
  out : Outport
  wires:
  in/1 -> Sum1/1, MinMax1/1, MinMax/1
  MinMax/1 -> Sum/1
  MinMax1/1 -> Sum/2
  Sum1/1 -> out/1
  Sum/1 -> Gain/1
  Gain/1 -> Scope/1, Sum1/2

== system Test_01/DFIG 2.0 MW 690 V/Control/Cancelation of cc ==
  note: Stator Flux
  note: Ωm rd/s
      | Mechanic
  note: ωs (Hz)
  note: Pole Pairs
  note: ωr = ωs - ωm
  note: ωs (rd/s)
  note: ωm (rd/s)
      | Electrical
  Vd : Inport
  Vq : Inport  Port=2
  omega_m (Ωm) : Inport  Port=3
  Constant : Constant  Value=f
  Constant1 : Constant  Value=Fs
  Fcn : Fcn  Expr=u[1]-u[5]*sigma*Lr*u[4]
  Fcn1 : Fcn  Expr=u[2]+u[5]*sigma*Lr*u[3]+u[5]*(Lm/Ls)*u[6]
  Gain : Gain  Gain=p
  Gain1 : Gain  Gain=2*pi
  Mux : Mux  Inputs=2
  Mux1 : Mux  Inputs=6
  Sum : Sum  Inputs=|+-
  Vdr  Vqr : Outport
  tag scope: omega_s=global, vdr=global, vqr=global
  wires:
  Mux/1 -> Vdr  Vqr/1
  Fcn/1 -> [vdr], Mux/1
  Fcn1/1 -> [vqr], Mux/2
  Vd/1 -> Mux1/1
  Vq/1 -> Mux1/2
  Mux1/1 -> Fcn1/1, Fcn/1
  [idr] -> Mux1/3
  [iqr] -> Mux1/4
  Constant1/1 -> Mux1/6
  omega_m (Ωm)/1 -> Gain/1
  Gain/1 -> Sum/2
  Constant/1 -> Gain1/1
  Gain1/1 -> [omega_s], Sum/1
  Sum/1 -> Mux1/5

== system Test_01/DFIG 2.0 MW 690 V/Control/PI Id ==
  idr_ref : Inport
  idr_means : Inport  Port=2
  Discrete-Time Integrator : DiscreteIntegrator  SampleTime=1/fsw  LimitOutput=on  UpperSaturationLimit=Vbus_ref/sqrt(3)  LowerSaturationLimit=-Vbus_ref/sqrt(3)  ICPrevOutput=DiscIntNeverNeededParam  ICPrevScaledInput=DiscIntNeverNeededParam
  Error : Display
  Gain : Gain  Gain=kp_id
  Gain1 : Gain  Gain=ki_id
  Mean : Display
  Mux : Mux  Inputs=3
  Ref : Display
  Sat : Display
  Sat2 : Display
  Saturation : Saturate  UpperLimit=Vbus_ref/sqrt(3)  LowerLimit=-Vbus_ref/sqrt(3)
  Scope : Scope
  Sum : Sum  Inputs=|+-
  Sum1 : Sum  Inputs=|++
  Vd : Outport
  wires:
  idr_means/1 -> Mean/1, Mux/2, Sum/2
  idr_ref/1 -> Ref/1, Mux/1, Sum/1
  Sum/1 -> Gain/1, Gain1/1, Mux/3, Error/1
  Gain/1 -> Sum1/1
  Gain1/1 -> Discrete-Time Integrator/1
  Discrete-Time Integrator/1 -> Sat2/1, Sum1/2
  Sum1/1 -> Saturation/1
  Saturation/1 -> Sat/1, Vd/1
  Mux/1 -> Scope/1

== system Test_01/DFIG 2.0 MW 690 V/Control/PI Iq ==
  iqr_ref : Inport
  iqr_means : Inport  Port=2
  Discrete-Time Integrator : DiscreteIntegrator  SampleTime=1/fsw  LimitOutput=on  UpperSaturationLimit=Vbus_ref/sqrt(3)  LowerSaturationLimit=-Vbus_ref/sqrt(3)  ICPrevOutput=DiscIntNeverNeededParam  ICPrevScaledInput=DiscIntNeverNeededParam
  Display1 : Display
  Error : Display
  Gain : Gain  Gain=kp_iq
  Gain1 : Gain  Gain=ki_iq
  Mean : Display
  Mux : Mux  Inputs=3
  Ref : Display
  Sat : Display
  Saturation : Saturate  UpperLimit=Vbus_ref/sqrt(3)  LowerLimit=-Vbus_ref/sqrt(3)
  Scope : Scope
  Sum : Sum  Inputs=|+-
  Sum1 : Sum  Inputs=|++
  Vq : Outport
  wires:
  Gain/1 -> Sum1/1
  Gain1/1 -> Discrete-Time Integrator/1
  Sum1/1 -> Saturation/1
  Discrete-Time Integrator/1 -> Display1/1, Sum1/2
  iqr_means/1 -> Sum/2, Mean/1, Mux/2
  iqr_ref/1 -> Sum/1, Ref/1, Mux/1
  Sum/1 -> Gain/1, Gain1/1, Mux/3, Error/1
  Saturation/1 -> Sat/1, Vq/1
  Mux/1 -> Scope/1

== system Test_01/DFIG 2.0 MW 690 V/Control/abc - α//β  ==
  note: iβr
  note: iαr
  iabcr : Inport
  Fcn : Fcn  Expr=2/3*(u[1]-u[2]/2-u[3]/2)
  Fcn1 : Fcn  Expr=2/3*(u[2]*(sqrt(3)/2)-u[3]*(sqrt(3)/2))
  Mux : Mux  Inputs=2
  i αr/βr : Outport
  wires:
  Mux/1 -> i αr/βr/1
  iabcr/1 -> Fcn1/1, Fcn/1
  Fcn/1 -> Mux/1
  Fcn1/1 -> Mux/2

== system Test_01/DFIG 2.0 MW 690 V/Control/d//q - α//β ==
  Vdr  Vqr : Inport
  theta_r (θr) : Inport  Port=2
  Fcn : Fcn  Expr=u(1)*cos(u[3])-u[2]*sin(u[3])
  Fcn1 : Fcn  Expr=u(1)*sin(u[3])+u[2]*cos(u[3])
  Mux : Mux  Inputs=2
  Mux1 : Mux  Inputs=2
  V αr/βr : Outport
  wires:
  Mux/1 -> V αr/βr/1
  Fcn/1 -> Mux/1
  Fcn1/1 -> Mux/2
  Vdr  Vqr/1 -> Mux1/1
  theta_r (θr)/1 -> Mux1/2
  Mux1/1 -> Fcn/1, Fcn1/1

== system Test_01/DFIG 2.0 MW 690 V/Control/α//β - abc ==
  V αr/βr : Inport
  Fcn : Fcn  Expr=u(1)
  Fcn1 : Fcn  Expr=-(u[1]/2)+u[2]*(sqrt(3)/2)
  Fcn2 : Fcn  Expr=-(u[1]/2)-u[2]*(sqrt(3)/2)
  Mux : Mux  Inputs=3
  Vabcr : Outport
  wires:
  Mux/1 -> Vabcr/1
  V αr/βr/1 -> Fcn2/1, Fcn1/1, Fcn/1
  Fcn/1 -> Mux/1
  Fcn1/1 -> Mux/2
  Fcn2/1 -> Mux/3

== system Test_01/DFIG 2.0 MW 690 V/Control/α//β - d//q ==
  i αr/βr : Inport
  theta_r (θr) : Inport  Port=2
  Fcn : Fcn  Expr=u(1)*cos(u[3])+u[2]*sin(u[3])
  Fcn1 : Fcn  Expr=-u(1)*sin(u[3])+u[2]*cos(u[3])
  Mux : Mux  Inputs=2
  Mux1 : Mux  Inputs=2
  i dr/qr : Outport
  wires:
  Mux/1 -> i dr/qr/1
  Fcn/1 -> Mux/1
  Fcn1/1 -> Mux/2
  i αr/βr/1 -> Mux1/1
  theta_r (θr)/1 -> Mux1/2
  Mux1/1 -> Fcn1/1, Fcn/1

== system Test_01/DFIG 2.0 MW 690 V/Control1/ Angle Rotor ==
  note: Vg α/β
  "Vabcg " : Inport
  " abc - αβ " : Subsystem
  Demux : Demux  Outputs=2
  θv=tan^(-1) (Vβ/Vα) : Trigonometry  Operator=atan2
  theta_g (θg) : Outport
  wires:
  " abc - αβ "/1("Vg α/β ") -> Demux/1
  Demux/1 -> θv=tan^(-1) (Vβ/Vα)/2
  Demux/2 -> θv=tan^(-1) (Vβ/Vα)/1
  "Vabcg "/1 -> " abc - αβ "/1(Vabcg)
  θv=tan^(-1) (Vβ/Vα)/1 -> theta_g (θg)/1

== system Test_01/DFIG 2.0 MW 690 V/Control1/3er Harmonic Inyection ==
  in : Inport
  Gain : Gain  Gain=-0.5
  MinMax : MinMax
  MinMax1 : MinMax  Function=max
  Scope : Scope
  Sum : Sum  Inputs=|++
  Sum1 : Sum  Inputs=|++
  out : Outport
  wires:
  Gain/1 -> Sum1/2, Scope/1
  Sum/1 -> Gain/1
  Sum1/1 -> out/1
  MinMax1/1 -> Sum/2
  MinMax/1 -> Sum/1
  in/1 -> MinMax/1, MinMax1/1, Sum1/1

== system Test_01/DFIG 2.0 MW 690 V/Control1/Cancelation of cc ==
  Id : Inport
  Iq : Inport  Port=2
  Display : Display
  Fcn : Fcn  Expr=u[1]-u[4]*Lg*(2*pi*f)
  Fcn1 : Fcn  Expr=u[2]+u[3]*Lg*(2*pi*f)
  Mux : Mux  Inputs=2
  Mux1 : Mux
  Vdg  Vqg : Outport
  tag scope: vdg=global, vqg=global
  wires:
  [iqg] -> Mux1/4
  [idg] -> Mux1/3
  Mux1/1 -> Fcn/1, Fcn1/1
  Iq/1 -> Mux1/2
  Id/1 -> Mux1/1
  Fcn1/1 -> Mux/2, [vqg]
  Fcn/1 -> Mux/1, Display/1, [vdg]
  Mux/1 -> Vdg  Vqg/1

== system Test_01/DFIG 2.0 MW 690 V/Control1/PI ==
  note: signal
  note: reference
  "ref Vbus " : Inport
  "means Vbus " : Inport  Port=2
  Discrete-Time Integrator1 : DiscreteIntegrator  SampleTime=1/fsw  LimitOutput=on  UpperSaturationLimit=Ps  LowerSaturationLimit=-Ps  ICPrevOutput=DiscIntNeverNeededParam  ICPrevScaledInput=DiscIntNeverNeededParam
  Error : Display
  Gain2 : Gain  Gain=kp_v
  Gain3 : Gain  Gain=ki_v
  Mean : Display
  Mux : Mux  Inputs=3
  Ref : Display
  Sat : Display
  Sat 1 : Display
  Saturation1 : Saturate  UpperLimit=Ps  LowerLimit=-Ps
  Scope : Scope
  Sum2 : Sum  Inputs=|+-
  Sum3 : Sum  Inputs=|++
  P_rotor_ref : Outport
  wires:
  Discrete-Time Integrator1/1 -> Sat 1/1, Sum3/2
  Gain3/1 -> Discrete-Time Integrator1/1
  Sum3/1 -> Saturation1/1
  Gain2/1 -> Sum3/1
  Saturation1/1 -> Sat/1, P_rotor_ref/1
  "means Vbus "/1 -> Sum2/2, Mean/1, Mux/2
  "ref Vbus "/1 -> Sum2/1, Ref/1, Mux/1
  Sum2/1 -> Gain2/1, Gain3/1, Mux/3, Error/1
  Mux/1 -> Scope/1

== system Test_01/DFIG 2.0 MW 690 V/Control1/PI Id ==
  idg_ref : Inport
  idg_means : Inport  Port=2
  Discrete-Time Integrator : DiscreteIntegrator  SampleTime=1/fsw  LimitOutput=on  UpperSaturationLimit=Vbus_ref/sqrt(3)*2  LowerSaturationLimit=-Vbus_ref/sqrt(3)*2  ICPrevOutput=DiscIntNeverNeededParam  ICPrevScaledInput=DiscIntNeverNeededParam
  Error : Display
  Gain : Gain  Gain=kp_idg
  Gain1 : Gain  Gain=ki_idg
  Mean : Display
  Mux : Mux  Inputs=3
  Ref : Display
  Sat : Display
  Sat 1 : Display
  Saturation : Saturate  UpperLimit=Vbus_ref/sqrt(3)*2  LowerLimit=-Vbus_ref/sqrt(3)*2
  Scope : Scope
  Sum : Sum  Inputs=|+-
  Sum1 : Sum  Inputs=|++
  out : Outport
  wires:
  Saturation/1 -> Sat/1, out/1
  Sum1/1 -> Saturation/1
  Discrete-Time Integrator/1 -> Sat 1/1, Sum1/2
  Gain1/1 -> Discrete-Time Integrator/1
  Gain/1 -> Sum1/1
  idg_means/1 -> Mean/1, Mux/2, Sum/2
  idg_ref/1 -> Ref/1, Mux/1, Sum/1
  Sum/1 -> Gain/1, Gain1/1, Mux/3, Error/1
  Mux/1 -> Scope/1

== system Test_01/DFIG 2.0 MW 690 V/Control1/PI Iq ==
  iqg_ref : Inport
  iqg_means : Inport  Port=2
  Discrete-Time Integrator : DiscreteIntegrator  SampleTime=1/fsw  LimitOutput=on  UpperSaturationLimit=Vbus_ref/sqrt(3)  LowerSaturationLimit=-Vbus_ref/sqrt(3)  ICPrevOutput=DiscIntNeverNeededParam  ICPrevScaledInput=DiscIntNeverNeededParam
  Error : Display
  Gain : Gain  Gain=kp_iqg
  Gain1 : Gain  Gain=ki_iqg
  Mean : Display
  Mux : Mux  Inputs=3
  Ref : Display
  Sat : Display
  Sat 1 : Display
  Saturation : Saturate  UpperLimit=Vbus_ref/sqrt(3)  LowerLimit=-Vbus_ref/sqrt(3)
  Scope : Scope
  Sum : Sum  Inputs=|+-
  Sum1 : Sum  Inputs=|++
  out : Outport
  wires:
  Sum1/1 -> Saturation/1
  Discrete-Time Integrator/1 -> Sat 1/1, Sum1/2
  Gain1/1 -> Discrete-Time Integrator/1
  Gain/1 -> Sum1/1
  Saturation/1 -> Sat/1, out/1
  iqg_means/1 -> Sum/2, Mean/1, Mux/2
  iqg_ref/1 -> Sum/1, Ref/1, Mux/1
  Sum/1 -> Mux/3, Error/1, Gain/1, Gain1/1
  Mux/1 -> Scope/1

== system Test_01/DFIG 2.0 MW 690 V/Control1/abc - α//β   ==
  note: iαg
  note: iβg
  iabcg : Inport
  Fcn : Fcn  Expr=2/3*(u[1]-u[2]/2-u[3]/2)
  Fcn1 : Fcn  Expr=2/3*(u[2]*(sqrt(3)/2)-u[3]*(sqrt(3)/2))
  Mux : Mux  Inputs=2
  i αg/βg : Outport
  wires:
  Fcn1/1 -> Mux/2
  Fcn/1 -> Mux/1
  iabcg/1 -> Fcn/1, Fcn1/1
  Mux/1 -> i αg/βg/1

== system Test_01/DFIG 2.0 MW 690 V/Control1/d//q  α//β  ==
  Vdg  Vqg : Inport
  theta_g (θg) : Inport  Port=2
  Fcn : Fcn  Expr=u(1)*cos(u[3])-u[2]*sin(u[3])
  Fcn1 : Fcn  Expr=u(1)*sin(u[3])+u[2]*cos(u[3])
  Mux : Mux  Inputs=2
  Mux1 : Mux  Inputs=2
  V αg/βg : Outport
  wires:
  Mux1/1 -> Fcn1/1, Fcn/1
  theta_g (θg)/1 -> Mux1/2
  Vdg  Vqg/1 -> Mux1/1
  Fcn1/1 -> Mux/2
  Fcn/1 -> Mux/1
  Mux/1 -> V αg/βg/1

== system Test_01/DFIG 2.0 MW 690 V/Control1/α//β - abc ==
  V αg/βg : Inport
  Fcn : Fcn  Expr=u(1)
  Fcn1 : Fcn  Expr=-(u[1]/2)+u[2]*(sqrt(3)/2)
  Fcn2 : Fcn  Expr=-(u[1]/2)-u[2]*(sqrt(3)/2)
  Mux : Mux  Inputs=3
  Vabcg : Outport
  wires:
  Fcn2/1 -> Mux/3
  Fcn1/1 -> Mux/2
  Fcn/1 -> Mux/1
  V αg/βg/1 -> Fcn/1, Fcn1/1, Fcn2/1
  Mux/1 -> Vabcg/1

== system Test_01/DFIG 2.0 MW 690 V/Control1/α//β - d//q ==
  i αg/βg : Inport
  theta_g (θg) : Inport  Port=2
  Fcn : Fcn  Expr=u(1)*cos(u[3])+u[2]*sin(u[3])
  Fcn1 : Fcn  Expr=-u(1)*sin(u[3])+u[2]*cos(u[3])
  Mux : Mux  Inputs=2
  Mux1 : Mux  Inputs=2
  i dg/qg : Outport
  wires:
  Mux1/1 -> Fcn/1, Fcn1/1
  theta_g (θg)/1 -> Mux1/2
  i αg/βg/1 -> Mux1/1
  Fcn1/1 -> Mux/2
  Fcn/1 -> Mux/1
  Mux/1 -> i dg/qg/1

== system Test_01/BESS 1.0 MW 690 V/Control System/ Angle Rotor/ abc - αβ  ==
  Vabc_bat : Inport
  Fcn : Fcn  Expr=2/3*(u[1]-u[2]/2-u[3]/2)
  Fcn1 : Fcn  Expr=2/3*(u[2]*(sqrt(3)/2)-u[3]*(sqrt(3)/2))
  Mux : Mux  Inputs=2
  "V α/β_bat " : Outport
  wires:
  Mux/1 -> "V α/β_bat "/1
  Vabc_bat/1 -> Fcn1/1, Fcn/1
  Fcn/1 -> Mux/1
  Fcn1/1 -> Mux/2

== system Test_01/DFIG 2.0 MW 690 V/Control/ Angle Rotor/Clarke: abc - αβ  ==
  Vabc : Inport
  Fcn : Fcn  Expr=2/3*(u[1]-u[2]/2-u[3]/2)
  Fcn1 : Fcn  Expr=2/3*(u[2]*(sqrt(3)/2)-u[3]*(sqrt(3)/2))
  Mux : Mux  Inputs=2
  "Vαs/βs " : Outport
  wires:
  Mux/1 -> "Vαs/βs "/1
  Vabc/1 -> Fcn1/1, Fcn/1
  Fcn/1 -> Mux/1
  Fcn1/1 -> Mux/2

== system Test_01/DFIG 2.0 MW 690 V/Control1/ Angle Rotor/ abc - αβ  ==
  Vabcg : Inport
  Fcn : Fcn  Expr=2/3*(u[1]-u[2]/2-u[3]/2)
  Fcn1 : Fcn  Expr=2/3*(u[2]*(sqrt(3)/2)-u[3]*(sqrt(3)/2))
  Mux : Mux  Inputs=2
  "Vg α/β " : Outport
  wires:
  Fcn1/1 -> Mux/2
  Fcn/1 -> Mux/1
  Vabcg/1 -> Fcn/1, Fcn1/1
  Mux/1 -> "Vg α/β "/1
